simulink model "controller_Harness_Selector"  (R2023b)
settings: Solver=FixedStepAuto  StartTime=0.0  StopTime=6  FixedStep=1/100  RelTol=1e-3
libraries: simulink x1
settings Model: Creator=Matteo  LastModifiedBy=dadog
settings OptimizationCC: ReuseModelBlockBuffer=off
settings DebuggingCC: SigSpecEnsureSampleTimeMsg=none  UnconnectedInputMsg=warning  UnconnectedOutputMsg=warning  UnconnectedLineMsg=warning
settings ModelReferenceCC: EnableRefExpFcnMdlSchedulingChecks=on
settings RTWCC: DLArmComputeVersion=19.05
settings ConfigComp: CovEnable=on  CovScope=Subsystem  RecordCoverage=on

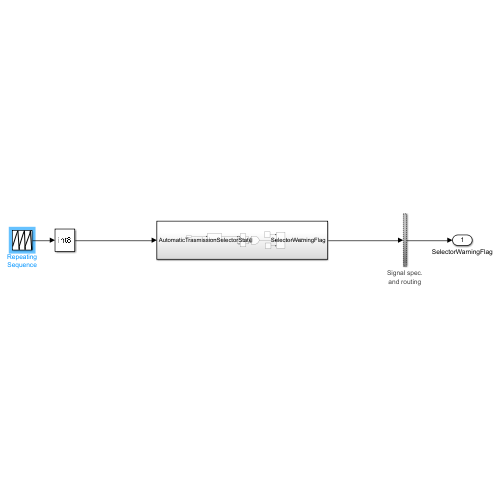
[thumbnail: Simulink's stored preview of the top-level diagram]
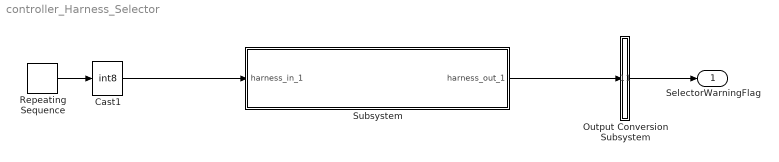
== system controller_Harness_Selector ==
  Cast1 : DataTypeConversion  OutDataTypeStr=int8  SaturateOnIntegerOverflow=off  RndMeth=Floor
  Output Conversion Subsystem : Subsystem  Tag=__SLT_OCS__  Description=|
      | Signal spec.
      | and routing
      settings: AttributesFormatString=%<Description>
  Repeating Sequence : simulink/Sources/Repeating Sequence  rep_seq_t=[0 4 5 6]  rep_seq_y=[0 4 5 -1]
  Subsystem : Subsystem  Tag=__SL_testing_harness_stub_
  SelectorWarningFlag : Outport
  wires:
  Repeating Sequence/1 -> Cast1/1
  Output Conversion Subsystem/1(Outport_1) -> SelectorWarningFlag/1
  Cast1/1 -> Subsystem/1(harness_in_1)
  Subsystem/1(harness_out_1) -> Output Conversion Subsystem/1(Inport_1)

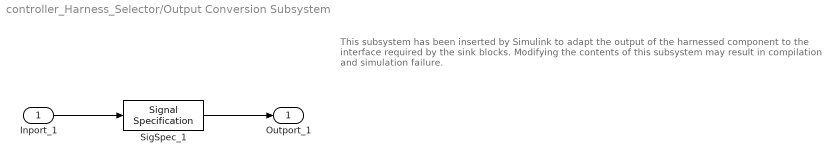
== system controller_Harness_Selector/Output Conversion Subsystem ==
  note: This subsystem has been inserted by Simulink to adapt the output of the harnessed component to the interface required by the sink blocks.
      |  Modifying the contents of this subsystem may result in compilation and simulation failure.
  Inport_1 : Inport
  SigSpec_1 : SignalSpecification  OutDataTypeStr=boolean  Dimensions=[1]  SampleTime=0.01
  Outport_1 : Outport
  wires:
  Inport_1/1 -> SigSpec_1/1
  SigSpec_1/1 -> Outport_1/1

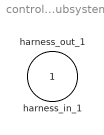
== system controller_Harness_Selector/Subsystem ==
  harness_in_1 : Inport
  harness_out_1 : Outport
